simulink model "modulation_final_1"  (R2018b)
settings: Solver=ode23  StartTime=0.0  StopTime=2  MaxStep=0.01725/4  RelTol=1e-3
values from neighbouring files (symbols this model uses):
  fs = 20000    [Motor_parameters_project.m]
  In = 189    [Motor_parameters_project.m]
  J = 0.0151    [Motor_parameters_project.m]
  Lm = 0.38e-3    (= 0.00038)    [Motor_parameters_project.m]
  Lr = Lm + Ldr    (= 0.00041116)    [Motor_parameters_project.m]
  Ls = Lm + Lds    (= 0.00041116)    [Motor_parameters_project.m]
  Omegae = 2*pi*fn    (= 364.424747816)    [Motor_parameters_project.m]
  p = 2.0    (= 2)    [Motor_parameters_project.m]
  Rr = 2.69e-3    (= 0.00269)    [Motor_parameters_project.m]
  Rs = 2.5e-3    (= 0.0025)    [Motor_parameters_project.m]
  T_rated = Pn/(2*pi*nn/60)    (= 30.0363631473)    [Motor_parameters_project.m]
  Udc = 36    [Motor_parameters_project.m]
  Un = 24    [Motor_parameters_project.m]
libraries: powerlib_meascontrol x1, powerlib x1
settings Model: Creator=estef  LastModifiedBy=faheem

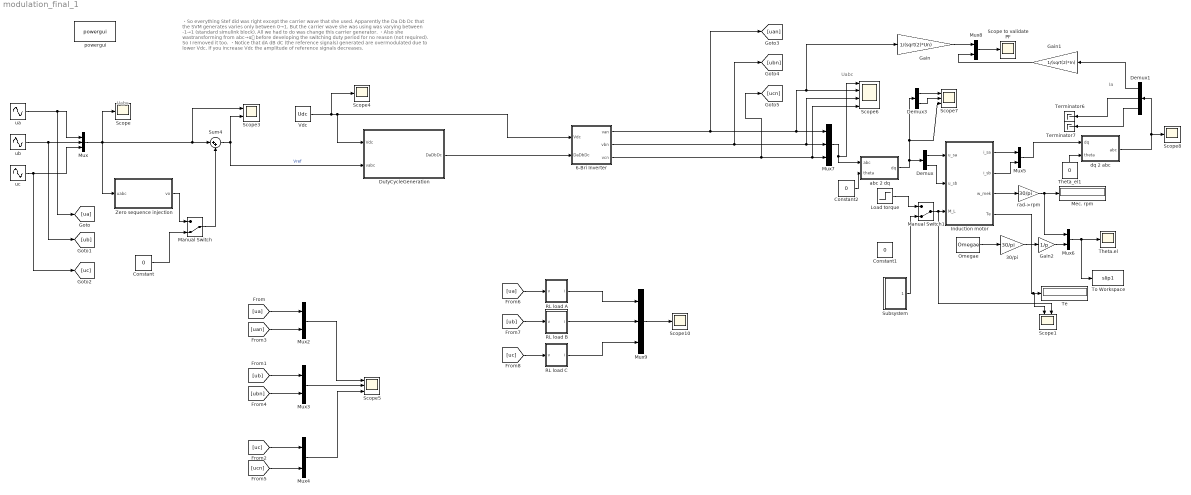
== system modulation_final_1 ==
  note: ・So everything  Stef did was right except the carrier wave that she used. Apparently the Da Db Dc that the SVM generates varies only between 0→1. But the
      | carrier wave she was using was varying between -1→1 (standard simulink block). All we had to do was change this carrier generator.
      | ・Also she wastransforming from abc→α🅱️ before developing the switching duty period for no reason (not required). So I removed it too.
      | ・Notice that dA dB dC (the reference signals) generated are overmodulated due to lower Vdc. If you increase Vdc the amplitude of reference signals decreases.
  note: Uabc
  note: Ia
  note: Uabc
  30/pi : Gain  Gain=30/pi
  6-Bri Inverter : Subsystem
  Constant : Constant  Value=0
  Constant1 : Constant  Value=0
  Constant2 : Constant  Value=0
  Demux : Demux  Outputs=2
  Demux1 : Demux  Outputs=3
  Demux3 : Demux  Outputs=2
  DutyCycleGeneration : Subsystem
  Gain : Gain  Gain=1/(sqrt(2)*Un)
  Gain1 : Gain  Gain=1/(sqrt(2)*In)
  Gain2 : Gain  Gain=1/p
  Induction motor : Subsystem
  Load torque : Step  Time=0.9  After=T_rated  SampleTime=0
  Manual Switch : ManualSwitch  CurrentSetting=0
  Manual Switch1 : ManualSwitch  CurrentSetting=0
  Mec. rpm : Display
  Mux : Mux  Inputs=3
  Mux{2..6,8} (6 alike) : Mux  Inputs=2
  Mux7 : Mux  Inputs=3
  Mux9 : Mux  Inputs=3
  Omegae : Constant  Value=Omegae
  RL load A : Subsystem
  RL load B : Subsystem
  RL load C : Subsystem
  Scope{,4,8,10} (4 alike) : Scope
  Scope to validate PF : Scope
  Scope1 : Scope  NumInputPorts=2
  Scope3 : Scope  NumInputPorts=2
  Scope5 : Scope  NumInputPorts=3
  Scope6 : Scope  NumInputPorts=4
  Scope7 : Scope  NumInputPorts=3
  Subsystem : Subsystem
  Sum4 : Sum  Inputs=|++
  Te : Display
  Terminator6 : Terminator
  Terminator7 : Terminator
  Theta.el : Scope
  Theta_el1 : Constant  Value=0
  To Workspace : ToWorkspace  VariableName=slip1  SaveFormat=Timeseries  SampleTime=-1
  "Vdc " : Constant  Value=Udc
  Zero sequence injection : Subsystem
  abc 2 dq : Subsystem
  dq 2 abc : Subsystem
  powergui : powerlib/powergui  Priority=1  SimulationMode=Continuous  SampleTime=0.0000001  frequency=60  Iterations=50  frequencyindice=60  Pbase=100e6  ErrMax=1e-4  UnitsV=kV  UnitsW=MW  buscounter=0  FunctionMessages=off  echomessages=off  EnableUseOfTLC=off  CurrentSourceSwitches=off  DisableSnubberDevices=off  DisableRonSwitches=off  DisableVfSwitches=off  DisplayEquations=off  SolverType=Tustin/Backward Euler (TBE)  Interpol=off  ExternalGateDelay=off  methode=off  Ts=100  x0status=blocks  SPID=off  SwTol=0  HookPort=off  RestoreLinks=warning  ResistiveCurrentMeasurement=off  Frange=[0:2:500]  Ylog=off  Xlog=on  ShowGrid=off  save=off  variable=ZData  structure=0  ZoomFFT=off  StartTime=0.0  cycles=1  DisplayStyle=1  fundamental=60  FreqAxis=off  MaxFrequency=1000  frequencyindicesteady=1  RmsSteady=1  display=off
  rad->rpm : Gain  Gain=30/pi  SaturateOnIntegerOverflow=on  OutDataTypeStr=Inherit: Same as input  ParamDataTypeStr=Inherit: Same as input
  ua : Sin  Amplitude=sqrt(2)*Un  Frequency=Omegae  SampleTime=0
  ub : Sin  Amplitude=sqrt(2)*Un  Frequency=Omegae  Phase=-2*pi/3  SampleTime=0
  uc : Sin  Amplitude=sqrt(2)*Un  Frequency=Omegae  Phase=2*pi/3  SampleTime=0
  wires:
  Sum4/1 -> DutyCycleGeneration/2(vabc), Scope3/2  "Vref"
  Mux/1 -> Scope/1, Scope3/1, Sum4/1, Zero sequence injection/1(uabc)
  Manual Switch/1 -> Sum4/2
  ub/1 -> Mux/2, [ub]
  Constant/1 -> Manual Switch/2
  ua/1 -> Mux/1, [ua]
  uc/1 -> Mux/3, [uc]
  Mux2/1 -> Scope5/1
  Mux3/1 -> Scope5/2
  Mux4/1 -> Scope5/3
  Zero sequence injection/1("vo ") -> Manual Switch/1
  [ua] -> Mux2/1
  [uan] -> Mux2/2
  [ubn] -> Mux3/2
  [ub] -> Mux3/1
  [ucn] -> Mux4/2
  [uc] -> Mux4/1
  Demux3/2 -> Scope7/2
  Load torque/1 -> Manual Switch1/1
  dq 2 abc/1(abc) -> Demux1/1, Scope8/1
  Omegae/1 -> 30/pi/1
  Mux8/1 -> Scope to validate PF/1
  Mux5/1 -> dq 2 abc/1(dq)
  Demux1/2 -> Terminator6/1
  Induction motor/3(w_mek) -> rad->rpm/1
  Induction motor/1(i_sa) -> Mux5/1
  Induction motor/2(i_sb) -> Mux5/2
  Gain/1 -> Mux8/1
  rad->rpm/1 -> Mux6/1, Mec. rpm/1
  Manual Switch1/1 -> Scope1/2, Induction motor/3(M_L)
  Demux1/1 -> Gain1/1
  Demux1/3 -> Terminator7/1
  Demux/2 -> Induction motor/2(u_sb)
  Gain1/1 -> Mux8/2
  30/pi/1 -> Gain2/1
  Mux6/1 -> To Workspace/1, Theta.el/1
  Demux3/1 -> Scope7/1
  Mux7/1 -> abc 2 dq/1(abc), Scope6/1
  Gain2/1 -> Mux6/2
  Induction motor/4(Te) -> Scope1/1, Te/1
  Demux/1 -> Induction motor/1(u_sa)
  abc 2 dq/1(dq) -> Scope7/3, Demux3/1, Demux/1
  Theta_el1/1 -> dq 2 abc/2(theta)
  RL load B/1(i) -> Mux9/2
  RL load C/1(i) -> Mux9/3
  RL load A/1(i) -> Mux9/1
  [ua] -> RL load A/1(v)
  [ub] -> RL load B/1(v)
  [uc] -> RL load C/1(v)
  6-Bri Inverter/1(van) -> Gain/1, Scope6/2, Mux7/1, [uan]
  6-Bri Inverter/2(vbn) -> Mux7/2, Scope6/3, [ubn]
  6-Bri Inverter/3(vcn) -> Mux7/3, Scope6/4, [ucn]
  Mux9/1 -> Scope10/1
  Constant2/1 -> abc 2 dq/2(theta)
  Subsystem/1(T_load) -> Manual Switch1/2
  "Vdc "/1 -> Scope4/1, 6-Bri Inverter/1(Vdc), DutyCycleGeneration/1(Vdc)
  DutyCycleGeneration/1(DaDbDc) -> 6-Bri Inverter/2(DaDbDc)

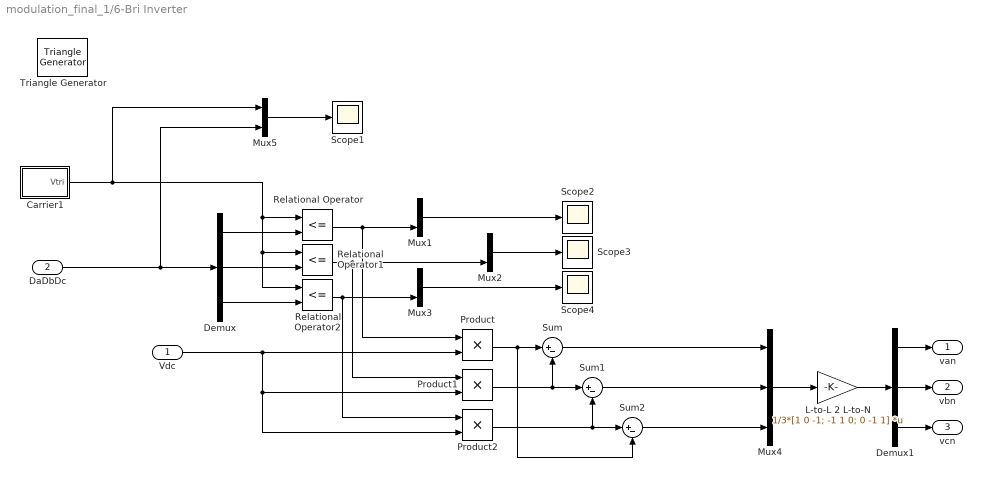
== system modulation_final_1/6-Bri Inverter ==
  Vdc : Inport
  DaDbDc : Inport  Port=2
  Carrier1 : Subsystem  mask{fsw=fs}
      mask prompts: fsw "switching frequency"
      mask init:
      | fsw2=fsw*2;
      | x=[0 1/4 3/4 1];
      | y=[0 -1     1    0];
      mask Display: plot([x  x+1 ],[y y])
  Demux : Demux  Outputs=3
  Demux1 : Demux  Outputs=3
  L-to-L 2 L-to-N : Gain  Gain=1/3*[1 0 -1; -1 1 0; 0 -1 1]  Multiplication=Matrix(K*u)
  Mux{1..3,5} (4 alike) : Mux  Inputs=2
  Mux4 : Mux  Inputs=3
  Product : Product  RndMeth=Zero
  Product1 : Product  RndMeth=Zero
  Product2 : Product  RndMeth=Zero
  Relational Operator : RelationalOperator  Operator=<=  RndMeth=Nearest
  Relational Operator1 : RelationalOperator  Operator=<=  RndMeth=Nearest
  Relational Operator2 : RelationalOperator  Operator=<=  RndMeth=Nearest
  Scope{1..4} (4 alike) : Scope
  Sum : Sum  Inputs=|+-
  Sum1 : Sum  Inputs=|+-
  Sum2 : Sum  Inputs=|+-
  Triangle Generator : powerlib_meascontrol/Pulse & Signal Generators/Triangle Generator  Freq=fs  Phase=90  Ts=0
  van : Outport
  vbn : Outport  Port=2
  vcn : Outport  Port=3
  wires:
  Demux/1 -> Relational Operator/2
  Mux1/1 -> Scope2/1
  Relational Operator/1 -> Mux1/2, Product/1
  Demux/2 -> Relational Operator1/2
  Demux/3 -> Relational Operator2/2
  Mux2/1 -> Scope3/1
  Mux3/1 -> Scope4/1
  Relational Operator1/1 -> Mux2/2, Product1/1
  Relational Operator2/1 -> Mux3/2, Product2/1
  Vdc/1 -> Product/2, Product1/2, Product2/2
  Product/1 -> Sum/1, Sum2/2
  Product1/1 -> Sum/2, Sum1/1
  Product2/1 -> Sum1/2, Sum2/1
  L-to-L 2 L-to-N/1 -> Demux1/1
  Mux4/1 -> L-to-L 2 L-to-N/1
  Sum/1 -> Mux4/1
  Sum2/1 -> Mux4/3
  Sum1/1 -> Mux4/2
  Demux1/1 -> van/1
  Demux1/2 -> vbn/1
  Demux1/3 -> vcn/1
  Mux5/1 -> Scope1/1
  ? -> Mux1/1
  Carrier1/1(Vtri) -> Mux5/1, Relational Operator/1, Relational Operator1/1, Relational Operator2/1
  DaDbDc/1 -> Mux5/2, Demux/1

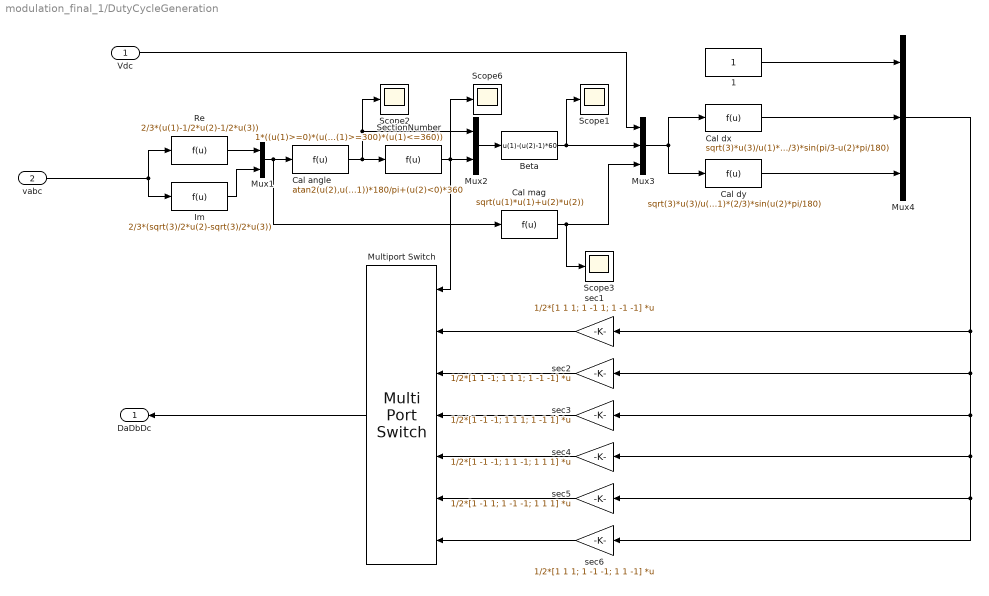
== system modulation_final_1/DutyCycleGeneration ==
  Vdc : Inport
  vabc : Inport  Port=2
  1 : Constant
  Beta : Fcn  Expr=u(1)-(u(2)-1)*60
  Cal angle : Fcn  Expr=atan2(u(2),u(1))*180/pi+(u(2)<0)*360
  Cal dx : Fcn  Expr=sqrt(3)*u(3)/u(1)*(2/3)*sin(pi/3-u(2)*pi/180)
  Cal dy : Fcn  Expr=sqrt(3)*u(3)/u(1)*(2/3)*sin(u(2)*pi/180)
  "Cal mag " : Fcn  Expr=sqrt(u(1)*u(1)+u(2)*u(2))
  Im : Fcn  Expr=2/3*(sqrt(3)/2*u(2)-sqrt(3)/2*u(3))
  Multiport Switch : MultiPortSwitch  Inputs=6
  Mux1 : Mux  Inputs=2
  Mux2 : Mux  Inputs=2
  Mux3 : Mux  Inputs=3
  Mux4 : Mux  Inputs=3
  Re : Fcn  Expr=2/3*(u(1)-1/2*u(2)-1/2*u(3))
  Scope{1..3,6} (4 alike) : Scope
  SectionNumber : Fcn  Expr=1*((u(1)>=0)*(u(1)<60))+2*((u(1)>=60)*(u(1)<120))+3*((u(1)>=120)*(u(1)<180))+4*((u(1)>=180)*(u(1)<240))+5*((u(1)>=240)*(u(1)<300))+6*((u(1)>=300)*(u(1)<=360))
  sec1 : Gain  Gain=1/2*[1 1 1; 1 -1 1; 1 -1 -1]  Multiplication=Matrix(K*u)
  sec2 : Gain  Gain=1/2*[1 1 -1; 1 1 1; 1 -1 -1]  Multiplication=Matrix(K*u)
  sec3 : Gain  Gain=1/2*[1 -1 -1; 1 1 1; 1 -1 1]  Multiplication=Matrix(K*u)
  sec4 : Gain  Gain=1/2*[1 -1 -1; 1 1 -1; 1 1 1]  Multiplication=Matrix(K*u)
  sec5 : Gain  Gain=1/2*[1 -1 1; 1 -1 -1; 1 1 1]  Multiplication=Matrix(K*u)
  sec6 : Gain  Gain=1/2*[1 1 1; 1 -1 -1; 1 1 -1]  Multiplication=Matrix(K*u)
  DaDbDc : Outport
  wires:
  Re/1 -> Mux1/1
  Im/1 -> Mux1/2
  Mux1/1 -> Cal angle/1, "Cal mag "/1
  Cal angle/1 -> SectionNumber/1, Mux2/1, Scope2/1
  SectionNumber/1 -> Mux2/2, Scope6/1, Multiport Switch/1
  Mux2/1 -> Beta/1
  Beta/1 -> Mux3/2, Scope1/1
  "Cal mag "/1 -> Mux3/3, Scope3/1
  Mux3/1 -> Cal dx/1, Cal dy/1
  Cal dx/1 -> Mux4/2
  Cal dy/1 -> Mux4/3
  Mux4/1 -> sec1/1, sec2/1, sec3/1, sec4/1, sec5/1, sec6/1
  sec1/1 -> Multiport Switch/2
  Multiport Switch/1 -> DaDbDc/1
  1/1 -> Mux4/1
  sec2/1 -> Multiport Switch/3
  sec3/1 -> Multiport Switch/4
  sec4/1 -> Multiport Switch/5
  sec5/1 -> Multiport Switch/6
  sec6/1 -> Multiport Switch/7
  vabc/1 -> Re/1, Im/1
  Vdc/1 -> Mux3/1

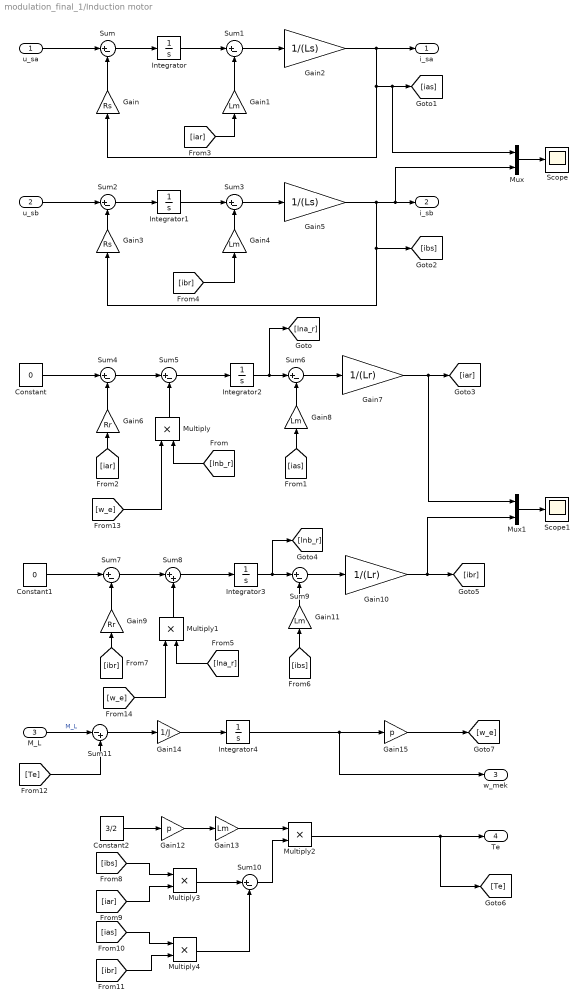
== system modulation_final_1/Induction motor ==
  u_sa : Inport
  u_sb : Inport  Port=2
  M_L : Inport  Port=3
  Constant : Constant  Value=0
  Constant1 : Constant  Value=0
  Constant2 : Constant  Value=3/2
  Gain : Gain  Gain=Rs
  Gain{1,4,8,11,13} (5 alike) : Gain  Gain=Lm
  Gain10 : Gain  Gain=1/(Lr)
  Gain12 : Gain  Gain=p
  Gain14 : Gain  Gain=1/J
  Gain15 : Gain  Gain=p
  Gain2 : Gain  Gain=1/(Ls)
  Gain3 : Gain  Gain=Rs
  Gain5 : Gain  Gain=1/(Ls)
  Gain6 : Gain  Gain=Rr
  Gain7 : Gain  Gain=1/(Lr)
  Gain9 : Gain  Gain=Rr
  Integrator{,1..4} (5 alike) : Integrator
  Multiply{,1..4} (5 alike) : Product
  Mux : Mux  Inputs=2
  Mux1 : Mux  Inputs=2
  Scope : Scope
  Scope1 : Scope
  Sum{,1..7,9..10} (10 alike) : Sum  Inputs=|+-
  Sum11 : Sum  Inputs=|-+
  Sum8 : Sum  Inputs=|++
  i_sa : Outport
  i_sb : Outport  Port=2
  w_mek : Outport  Port=3
  Te : Outport  Port=4
  wires:
  u_sa/1 -> Sum/1
  Gain/1 -> Sum/2
  Sum/1 -> Integrator/1
  Integrator/1 -> Sum1/1
  Gain1/1 -> Sum1/2
  Sum1/1 -> Gain2/1
  Gain2/1 -> Mux/1, [ias], Gain/1, i_sa/1
  Gain3/1 -> Sum2/2
  u_sb/1 -> Sum2/1
  Sum3/1 -> Gain5/1
  Gain4/1 -> Sum3/2
  Gain5/1 -> Mux/2, i_sb/1, [ibs], Gain3/1
  Sum2/1 -> Integrator1/1
  Integrator1/1 -> Sum3/1
  Constant/1 -> Sum4/1
  Gain6/1 -> Sum4/2
  Sum4/1 -> Sum5/1
  [lnb_r] -> Multiply/2
  Sum5/1 -> Integrator2/1
  Gain8/1 -> Sum6/2
  [ias] -> Gain8/1
  Integrator2/1 -> [lna_r], Sum6/1
  Sum6/1 -> Gain7/1
  Multiply/1 -> Sum5/2
  Gain7/1 -> Mux1/1, [iar]
  [iar] -> Gain6/1
  [ibr] -> Gain4/1
  [iar] -> Gain1/1
  Gain11/1 -> Sum9/2
  [ibr] -> Gain9/1
  [ibs] -> Gain11/1
  Multiply1/1 -> Sum8/2
  Integrator3/1 -> [lnb_r], Sum9/1
  Sum7/1 -> Sum8/1
  [lna_r] -> Multiply1/2
  Gain9/1 -> Sum7/2
  Sum9/1 -> Gain10/1
  Sum8/1 -> Integrator3/1
  Constant1/1 -> Sum7/1
  Gain13/1 -> Multiply2/1
  Sum10/1 -> Multiply2/2
  [ibs] -> Multiply3/1
  [iar] -> Multiply3/2
  Multiply3/1 -> Sum10/1
  [ias] -> Multiply4/1
  [ibr] -> Multiply4/2
  Multiply4/1 -> Sum10/2
  Constant2/1 -> Gain12/1
  Gain12/1 -> Gain13/1
  Multiply2/1 -> [Te], Te/1
  [Te] -> Sum11/2
  M_L/1 -> Sum11/1  "M_L"
  Sum11/1 -> Gain14/1
  Gain14/1 -> Integrator4/1
  Integrator4/1 -> Gain15/1, w_mek/1
  Gain15/1 -> [w_e]
  [w_e] -> Multiply/1
  [w_e] -> Multiply1/1
  Mux/1 -> Scope/1
  Mux1/1 -> Scope1/1
  Gain10/1 -> Mux1/2, [ibr]

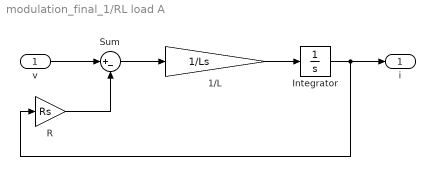
== system modulation_final_1/RL load A ==
  v : Inport
  1/L : Gain  Gain=1/Ls
  Integrator : Integrator
  R : Gain  Gain=Rs
  Sum : Sum  Inputs=|+-
  i : Outport
  wires:
  R/1 -> Sum/2
  Sum/1 -> 1/L/1
  1/L/1 -> Integrator/1
  Integrator/1 -> R/1, i/1
  v/1 -> Sum/1

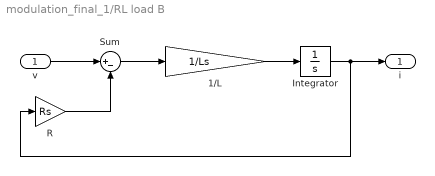
== system modulation_final_1/RL load B ==
  v : Inport
  1/L : Gain  Gain=1/Ls
  Integrator : Integrator
  R : Gain  Gain=Rs
  Sum : Sum  Inputs=|+-
  i : Outport
  wires:
  v/1 -> Sum/1
  Integrator/1 -> i/1, R/1
  1/L/1 -> Integrator/1
  Sum/1 -> 1/L/1
  R/1 -> Sum/2

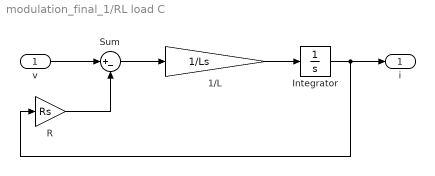
== system modulation_final_1/RL load C ==
  v : Inport
  1/L : Gain  Gain=1/Ls
  Integrator : Integrator
  R : Gain  Gain=Rs
  Sum : Sum  Inputs=|+-
  i : Outport
  wires:
  v/1 -> Sum/1
  Integrator/1 -> i/1, R/1
  1/L/1 -> Integrator/1
  Sum/1 -> 1/L/1
  R/1 -> Sum/2

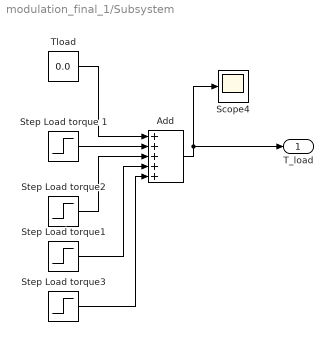
== system modulation_final_1/Subsystem ==
  Add : Sum  Inputs=+++++
  Scope4 : Scope
  Step Load torque 1 : Step  Time=0.9  After=5  SampleTime=0
  Step Load torque1 : Step  Time=1.5  After=7  SampleTime=0
  Step Load torque2 : Step  Time=1.2  After=8  SampleTime=0
  Step Load torque3 : Step  Time=1.8  After=10  SampleTime=0
  Tload : Constant  Value=0.0
  T_load : Outport
  wires:
  Add/1 -> T_load/1, Scope4/1
  Step Load torque 1/1 -> Add/2
  Tload/1 -> Add/1
  Step Load torque2/1 -> Add/3
  Step Load torque1/1 -> Add/4
  Step Load torque3/1 -> Add/5

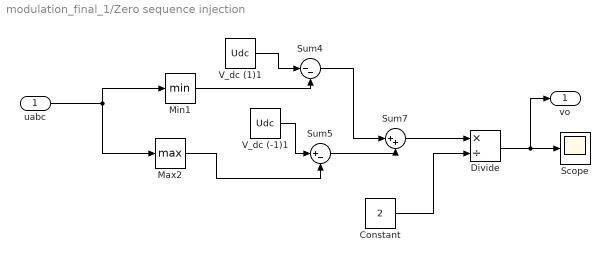
== system modulation_final_1/Zero sequence injection ==
  uabc : Inport
  Constant : Constant  Value=2
  Divide : Product  Inputs=*/
  Max2 : MinMax  Function=max
  Min1 : MinMax
  Scope : Scope
  Sum4 : Sum  Inputs=|--
  Sum5 : Sum  Inputs=|+-
  Sum7 : Sum  Inputs=|++
  V_dc (-1)1 : Constant  Value=Udc
  V_dc (1)1 : Constant  Value=Udc
  "vo " : Outport
  wires:
  Sum4/1 -> Sum7/1
  Sum7/1 -> Divide/1
  V_dc (-1)1/1 -> Sum5/1
  Min1/1 -> Sum4/2
  Constant/1 -> Divide/2
  Sum5/1 -> Sum7/2
  V_dc (1)1/1 -> Sum4/1
  Max2/1 -> Sum5/2
  uabc/1 -> Max2/1, Min1/1
  Divide/1 -> "vo "/1, Scope/1

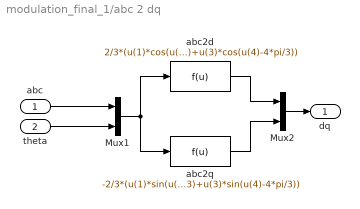
== system modulation_final_1/abc 2 dq ==
  abc : Inport
  theta : Inport  Port=2
  Mux1 : Mux  Inputs=2
  Mux2 : Mux  Inputs=2
  abc2d : Fcn  Expr=2/3*(u(1)*cos(u(4))+u(2)*cos(u(4)-2*pi/3)+u(3)*cos(u(4)-4*pi/3))
  abc2q : Fcn  Expr=-2/3*(u(1)*sin(u(4))+u(2)*sin(u(4)-2*pi/3)+u(3)*sin(u(4)-4*pi/3))
  dq : Outport
  wires:
  abc/1 -> Mux1/1
  theta/1 -> Mux1/2
  Mux1/1 -> abc2d/1, abc2q/1
  abc2d/1 -> Mux2/1
  abc2q/1 -> Mux2/2
  Mux2/1 -> dq/1

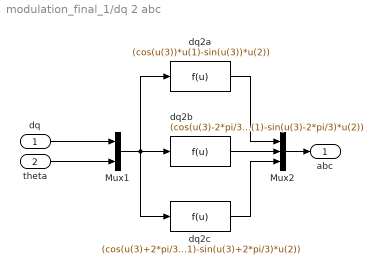
== system modulation_final_1/dq 2 abc ==
  dq : Inport
  theta : Inport  Port=2
  Mux1 : Mux  Inputs=2
  Mux2 : Mux  Inputs=3
  dq2a : Fcn  Expr=(cos(u(3))*u(1)-sin(u(3))*u(2))
  dq2b : Fcn  Expr=(cos(u(3)-2*pi/3)*u(1)-sin(u(3)-2*pi/3)*u(2))
  dq2c : Fcn  Expr=(cos(u(3)+2*pi/3)*u(1)-sin(u(3)+2*pi/3)*u(2))
  abc : Outport
  wires:
  Mux2/1 -> abc/1
  dq2b/1 -> Mux2/2
  dq2a/1 -> Mux2/1
  Mux1/1 -> dq2a/1, dq2c/1, dq2b/1
  theta/1 -> Mux1/2
  dq/1 -> Mux1/1
  dq2c/1 -> Mux2/3

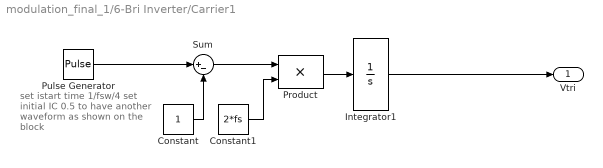
== system modulation_final_1/6-Bri Inverter/Carrier1 ==
  note: set istart time 1/fsw/4
      | set initial IC 0.5
      | to have another waveform
      |  as shown on the block
  Constant : Constant
  Constant1 : Constant  Value=2*fs
  Integrator1 : Integrator
  Product : Product  SaturateOnIntegerOverflow=on  OutDataTypeStr=Inherit: Same as first input
  Pulse Generator : DiscretePulseGenerator  PulseType=Time based  Amplitude=2  Period=1/fsw  PulseWidth=50
  Sum : Sum  Inputs=|+-  SaturateOnIntegerOverflow=on
  Vtri : Outport  InitialOutput=0
  wires:
  Pulse Generator/1 -> Sum/1
  Constant/1 -> Sum/2
  Sum/1 -> Product/1
  Constant1/1 -> Product/2
  Product/1 -> Integrator1/1
  Integrator1/1 -> Vtri/1
